simulink model "phase2_DOFBservo_notravel_simulation"  (R2018a)
settings: Solver=ode1  StartTime=0.0  StopTime=60  FixedStep=0.002  RelTol=1e-3  EnableMultiTasking=on
values from neighbouring files (symbols this model uses):
  A = [0 0 0 1 0 0 0 0 ... (first row only)    [q4.m]    (also in q5.m; q6.m; q7.m; q8.m)
  Apitch = [ ... (first row only)    [q4.m]    (also in q5.m; q6.m; q7.m; q8.m)
  Aroll = [ ... (first row only)    [q4.m]    (also in q5.m; q6.m; q7.m; q8.m)
  B = [0   0 ... (first row only)    [q4.m]    (also in q5.m; q6.m; q7.m; q8.m)
  Bpitch = [0;0;540]    [q4.m]    (also in q5.m; q6.m; q7.m; q8.m)
  Broll = [0;0;780]    [q4.m]    (also in q5.m; q6.m; q7.m; q8.m)
  C = [1 0 0 0 0 0 0 0 ... (first row only)    [q4.m]    (also in q5.m; q6.m; q7.m; q8.m)
  Cpitch = [1 0 0]    [q4.m]    (also in q5.m; q6.m; q7.m; q8.m)
  Croll = [1 0 0]    [q4.m]    (also in q5.m; q6.m; q7.m; q8.m)
  KIpitch = Kpitch(4)    [q9.m]
  KIroll = Kroll(4)    [q9.m]
  Kpitch = Kpitch(1:3)    [q9.m]
  Kroll = Kroll(1:3)    [q9.m]
  Lpitch = lqr(Apitch',Cpitch',Bpitch*Rww_pitch*Bpitch',Rvv_pitch)'    [q6.m]
  Lroll = lqr(Aroll',Croll',Broll*Rww_roll*Broll',Rvv_roll)'    [q6.m]
  Rpitch = [Rpitch; 0; 0]    [q9.m]
  Rroll = 0.02*eye(size(Broll,2))    [q4.m]    (also in q9.m = [Rroll; 0; 0])
libraries: simulink_extras x5
settings Model: ExtModeTrigDuration=51000  Creator=jeff  LastModifiedBy=NotCosmo
settings SolverCC: PositivePriorityOrder=on
settings DataIOCC: LimitDataPoints=on  SaveFormat=Array
settings OptimizationCC: InitFltsAndDblsToZero=on  LifeSpan=inf
settings DebuggingCC: SolverPrmCheckMsg=warning  SFUnexpectedBacktrackingDiag=warning  SFNoUnconditionalDefaultTransitionDiag=warning  SFExecutionAtInitializationDiag=none
settings HardwareCC: ProdBitPerPointer=32  ProdBitPerSizeT=32  ProdBitPerPtrDiffT=32  ProdLargestAtomicFloat=None  ProdIntDivRoundTo=Undefined  ProdEndianess=Unspecified  ProdWordSize=32  ProdHWDeviceType=32-bit Generic
settings ModelReferenceCC: PropagateSignalLabelsOutOfModel=off
settings RTWCC: SystemTargetFile=quarc_win64.tlc  TemplateMakefile=quarc_default_tmf  Description=QUARC Win64 Target
settings CodeAppCC: StateflowObjectComments=on
settings STFCustomTargetCC: TargetPreCompLibLocation=C:\PROGRA~3\QUARC\lib\2014a\win64\release  ConcurrentExecutionCompliant=on  GeneratePreprocessorConditionals=Disable all  SystemTargetFile=quarc_win64.tlc
settings GRTTargetCC: TargetPreCompLibLocation=C:\PROGRA~3\QUARC\lib\2014a\win64\release  TargetLangStandard=C89/C90 (ANSI)  ParMdlRefBuildCompliant=off  CompOptLevelCompliant=off  GeneratePreprocessorConditionals=Disable all  CombineOutputUpdateFcns=off  MatFileLogging=off  CPPClassGenCompliant=off  GRTInterface=on  UseToolchainInfoCompliant=off  ExtMode=on  ExtModeMexFile=quarc_comm
settings ConfigComp: CovMetricSettings=dw  CovHtmlReporting=on  CovSaveCumulativeToWorkspaceVar=on  CovSaveSingleToWorkspaceVar=on  CovExternalEMLEnable=off  CovSFcnEnable=off

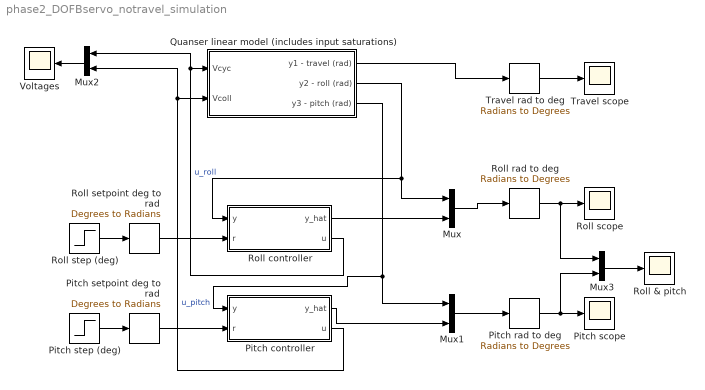
== system phase2_DOFBservo_notravel_simulation ==
  Mux{,1..3} (4 alike) : Mux  Inputs=2
  Pitch controller : Subsystem
  Pitch rad to deg : simulink_extras/Transformations/Radians to Degrees
  Pitch scope : Scope
  Pitch setpoint deg to rad : simulink_extras/Transformations/Degrees to Radians
  Pitch step (deg) : Step  Time=0  After=10  SampleTime=0
  Quanser linear model (includes input saturations) : Subsystem
  Roll & pitch : Scope
  Roll controller : Subsystem
  Roll rad to deg : simulink_extras/Transformations/Radians to Degrees
  Roll scope : Scope
  Roll setpoint deg to rad : simulink_extras/Transformations/Degrees to Radians
  Roll step (deg) : Step  Time=0  After=20  SampleTime=0
  Travel rad to deg : simulink_extras/Transformations/Radians to Degrees
  Travel scope : Scope
  "Voltages " : Scope
  wires:
  Quanser linear model (includes input saturations)/2(y2 - roll (rad)) -> Roll controller/1(y), Mux/1
  Roll controller/1(y_hat) -> Mux/2
  Mux/1 -> Roll rad to deg/1
  Roll rad to deg/1 -> Mux3/1, Roll scope/1
  Pitch setpoint deg to rad/1 -> Pitch controller/2(r)
  Pitch rad to deg/1 -> Mux3/2, Pitch scope/1
  Mux1/1 -> Pitch rad to deg/1
  Pitch controller/1(y_hat) -> Mux1/2
  Quanser linear model (includes input saturations)/3(y3 - pitch (rad)) -> Mux1/1, Pitch controller/1(y)
  Roll controller/2(u) -> Mux2/1, Quanser linear model (includes input saturations)/1(Vcyc)  "u_roll"
  Pitch controller/2(u) -> Mux2/2, Quanser linear model (includes input saturations)/2(Vcoll)  "u_pitch"
  Roll step (deg)/1 -> Roll setpoint deg to rad/1
  Travel rad to deg/1 -> Travel scope/1
  Quanser linear model (includes input saturations)/1(y1 - travel (rad)) -> Travel rad to deg/1
  Roll setpoint deg to rad/1 -> Roll controller/2(r)
  Pitch step (deg)/1 -> Pitch setpoint deg to rad/1
  Mux2/1 -> "Voltages "/1
  Mux3/1 -> Roll & pitch/1

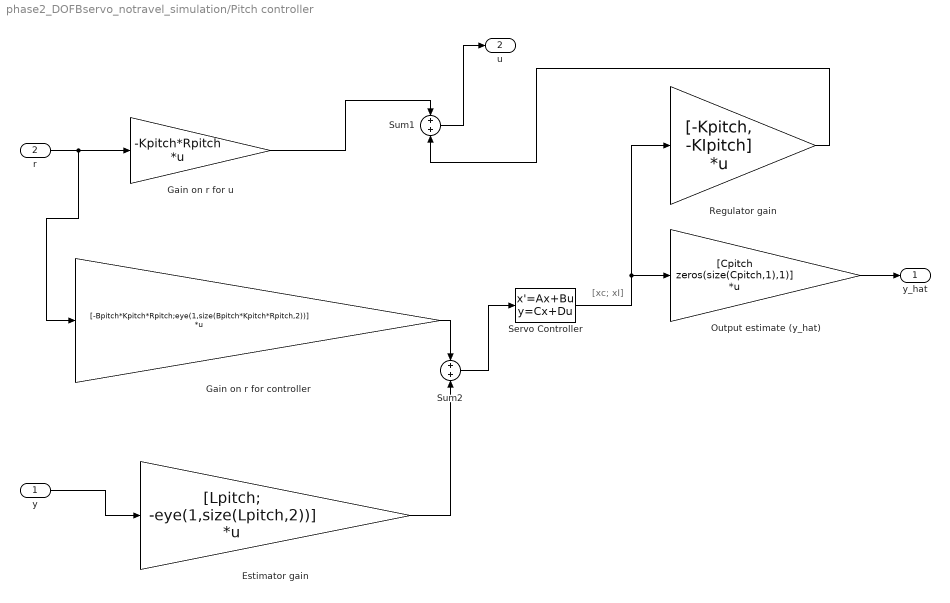
== system phase2_DOFBservo_notravel_simulation/Pitch controller ==
  note: [xc; xI]
  y : Inport
  r : Inport  Port=2
  Estimator gain : Gain  Gain=[Lpitch; -eye(1,size(Lpitch,2))]  Multiplication=Matrix(K*u)
  Gain on r for controller : Gain  Gain=[-Bpitch*Kpitch*Rpitch;eye(1,size(Bpitch*Kpitch*Rpitch,2))]  Multiplication=Matrix(K*u)
  Gain on r for u : Gain  Gain=-Kpitch*Rpitch  Multiplication=Matrix(K*u)
  Output estimate (y_hat) : Gain  Gain=[Cpitch zeros(size(Cpitch,1),1)]  Multiplication=Matrix(K*u)
  Regulator gain : Gain  Gain=[-Kpitch, -KIpitch]  Multiplication=Matrix(K*u)
  Servo Controller : StateSpace  A=[[Apitch-Lpitch*Cpitch-Bpitch*Kpitch] [-Bpitch*KIpitch]; zeros(1,size(Apitch,2)) zeros(1,size(Bpitch*KIpitch,2))]  B=eye(size(Apitch)+1)  C=eye(size(Apitch)+1)  D=zeros(size(Apitch)+1)  InitialCondition=[deg2rad(-5) 0 0 0]
  Sum1 : Sum  Inputs=+|+
  Sum2 : Sum  Inputs=+|+
  y_hat : Outport
  u : Outport  Port=2
  wires:
  Servo Controller/1 -> Regulator gain/1, Output estimate (y_hat)/1
  r/1 -> Gain on r for controller/1, Gain on r for u/1
  y/1 -> Estimator gain/1
  Output estimate (y_hat)/1 -> y_hat/1
  Gain on r for u/1 -> Sum1/1
  Gain on r for controller/1 -> Sum2/1
  Estimator gain/1 -> Sum2/2
  Sum2/1 -> Servo Controller/1
  Regulator gain/1 -> Sum1/2
  Sum1/1 -> u/1

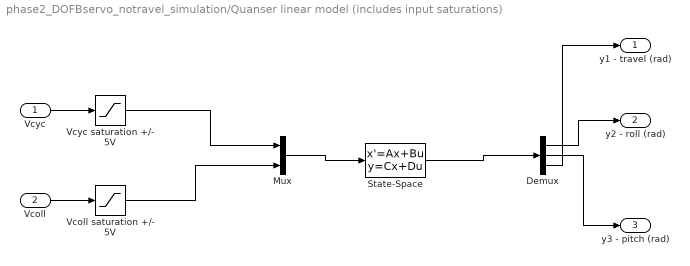
== system phase2_DOFBservo_notravel_simulation/Quanser linear model (includes input saturations) ==
  Vcyc : Inport
  Vcoll : Inport  Port=2
  Demux : Demux  Outputs=3
  Mux : Mux  Inputs=2
  State-Space : StateSpace  A=A  B=B  C=C  D=zeros(3,2)  InitialCondition=0
  Vcoll saturation +/- 5V : Saturate  UpperLimit=5.0  LowerLimit=-5.0
  Vcyc saturation +/- 5V : Saturate  UpperLimit=5.0  LowerLimit=-5.0
  y1 - travel (rad) : Outport
  y2 - roll (rad) : Outport  Port=2
  y3 - pitch (rad) : Outport  Port=3
  wires:
  Vcoll/1 -> Vcoll saturation +/- 5V/1
  Vcoll saturation +/- 5V/1 -> Mux/2
  Vcyc/1 -> Vcyc saturation +/- 5V/1
  Vcyc saturation +/- 5V/1 -> Mux/1
  Demux/1 -> y2 - roll (rad)/1
  Demux/2 -> y3 - pitch (rad)/1
  Demux/3 -> y1 - travel (rad)/1
  State-Space/1 -> Demux/1
  Mux/1 -> State-Space/1

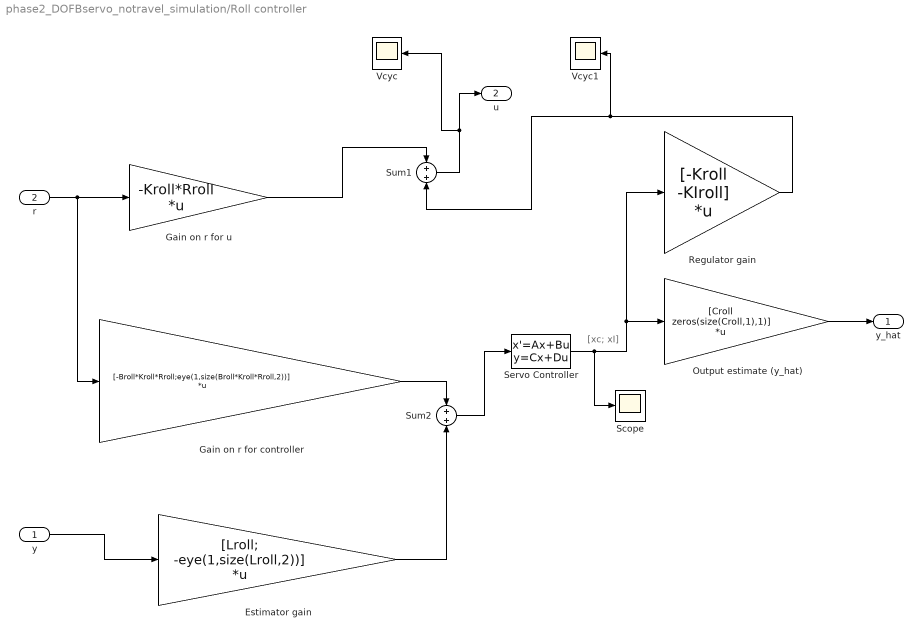
== system phase2_DOFBservo_notravel_simulation/Roll controller ==
  note: [xc; xI]
  y : Inport
  r : Inport  Port=2
  Estimator gain : Gain  Gain=[Lroll; -eye(1,size(Lroll,2))]  Multiplication=Matrix(K*u)
  Gain on r for controller : Gain  Gain=[-Broll*Kroll*Rroll;eye(1,size(Broll*Kroll*Rroll,2))]  Multiplication=Matrix(K*u)
  Gain on r for u : Gain  Gain=-Kroll*Rroll  Multiplication=Matrix(K*u)
  Output estimate (y_hat) : Gain  Gain=[Croll zeros(size(Croll,1),1)]  Multiplication=Matrix(K*u)
  Regulator gain : Gain  Gain=[-Kroll -KIroll]  Multiplication=Matrix(K*u)
  Scope : Scope
  Servo Controller : StateSpace  A=[[Aroll-Lroll*Croll-Broll*Kroll] [-Broll*KIroll]; zeros(1,size(Aroll,2)) zeros(1,size(Broll*KIroll,2))]  B=eye(size(Aroll)+1)  C=eye(size(Aroll)+1)  D=zeros(size(Aroll)+1)  InitialCondition=[deg2rad(0) 0 0 0]
  Sum1 : Sum  Inputs=+|+
  Sum2 : Sum  Inputs=+|+
  Vcyc : Scope
  Vcyc1 : Scope
  y_hat : Outport
  u : Outport  Port=2
  wires:
  Servo Controller/1 -> Scope/1, Regulator gain/1, Output estimate (y_hat)/1
  r/1 -> Gain on r for controller/1, Gain on r for u/1
  y/1 -> Estimator gain/1
  Output estimate (y_hat)/1 -> y_hat/1
  Gain on r for u/1 -> Sum1/1
  Gain on r for controller/1 -> Sum2/1
  Estimator gain/1 -> Sum2/2
  Sum2/1 -> Servo Controller/1
  Regulator gain/1 -> Vcyc1/1, Sum1/2
  Sum1/1 -> Vcyc/1, u/1
